simulink model "subscriber"  (Simulink 9.0)
settings: Solver=VariableStepAuto  StartTime=0.0  StopTime=inf  RelTol=1e-3
libraries: robotlib x1
settings Model: Creator=jonat  LastModifiedBy=jonat
settings DataIOCC: SaveFormat=Dataset
settings OptimizationCC: LifeSpan=auto
settings DebuggingCC: UnderspecifiedInitializationDetection=Simplified  MergeDetectMultiDrivingBlocksExec=error  SFUnexpectedBacktrackingDiag=error  SFNoUnconditionalDefaultTransitionDiag=error  SFExecutionAtInitializationDiag=warning
settings HardwareCC: ProdBitPerPointer=64  ProdBitPerSizeT=64  ProdBitPerPtrDiffT=64  ProdLargestAtomicFloat=Float  ProdIntDivRoundTo=Zero  ProdEndianess=LittleEndian  ProdWordSize=64  ProdHWDeviceType=Intel->x86-64 (Windows64)
settings ModelReferenceCC: PropagateSignalLabelsOutOfModel=on
settings CodeAppCC: StateflowObjectComments=off
settings GRTTargetCC: TargetLangStandard=C99 (ISO)
settings ConfigComp: CovMetricSettings=dwe  CovHtmlReporting=off  CovSaveCumulativeToWorkspaceVar=off  CovSaveSingleToWorkspaceVar=off  CovExternalEMLEnable=on

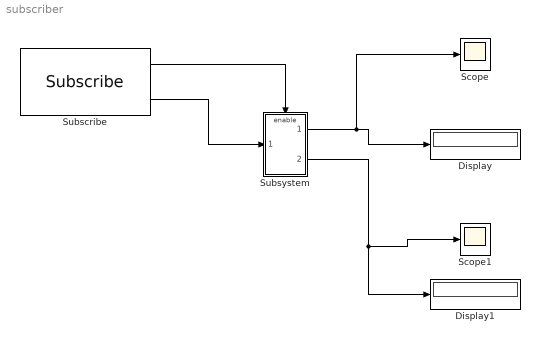
== system subscriber ==
  Display : Display
  Display1 : Display
  Scope : Scope
  Scope1 : Scope
  Subscribe : robotlib/Subscribe  SourceLibraryInfo=This block requires Robotics System Toolbox  topicSource=Select from ROS network  topic=/position  messageType=geometry_msgs/Twist  sampleTime=-1  messageQueueLength=1
      settings: SourceProductBaseCode=RO
  Subsystem : Subsystem
  wires:
  Subscribe/1 -> Subsystem/Enable
  Subscribe/2 -> Subsystem/1(In1)
  Subsystem/2(Out2) -> Scope1/1, Display1/1
  Subsystem/1(Out1) -> Scope/1, Display/1

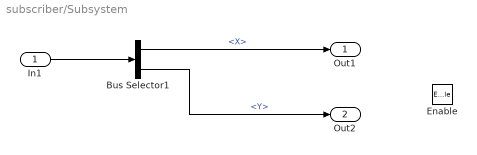
== system subscriber/Subsystem ==
  In1 : Inport
  Enable : EnablePort
  Bus Selector1 : BusSelector  DialogController=Simulink.DDGSource_BusSelector  OutputSignals=Linear.X,Linear.Y
  Out1 : Outport
  Out2 : Outport  Port=2
  wires:
  Bus Selector1/2 -> Out2/1  "<Y>"
  Bus Selector1/1 -> Out1/1  "<X>"
  In1/1 -> Bus Selector1/1
